simulink model "ringBufferPitchV2"  (R2021a)
settings: Solver=VariableStepAuto  StartTime=0.0  StopTime=10.0  RelTol=1e-3
libraries: hdlsllib x2
settings Model: Creator=Connor Watz  LastModifiedBy=Connor Watz

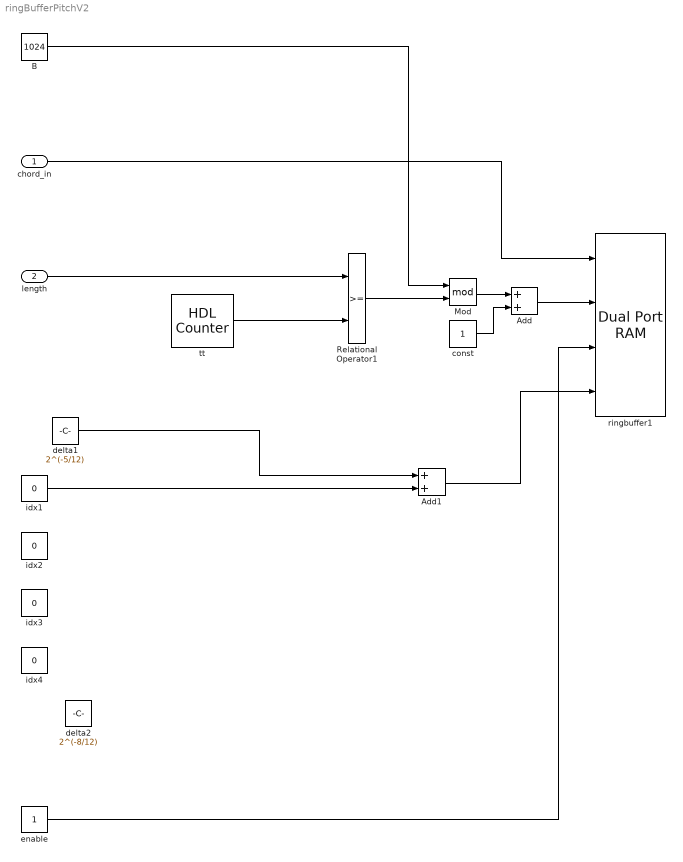
== system ringBufferPitchV2 ==
  chord_in : Inport
  length : Inport  Port=2
  Add : Sum
  Add1 : Sum
  B : Constant  Value=1024  SampleTime=-1
  Mod : Math  Operator=mod  SaturateOnIntegerOverflow=on
  Relational Operator1 : RelationalOperator  OutDataTypeStr=boolean  RndMeth=Nearest
  const : Constant
  delta1 : Constant  Value=2^(-5/12)
  delta2 : Constant  Value=2^(-8/12)
  enable : Constant
  idx{1..4} (4 alike) : Constant  Value=0
  ringbuffer1 : hdlsllib/HDL RAMs/Dual Port RAM  ram_size=8
      settings: SourceProductBaseCode=SL
  tt : hdlsllib/Sources/HDL Counter  CountType=Count limited  CountInit=0  CountStep=1  CountMax=25  CountFromType=Initial value  CountFrom=0  CountResetPort=off  CountLoadPort=off  CountEnbPort=off  CountDirPort=off  CountHitOutputPort=off  CountDataType=Unsigned  CountWordLen=8  CountFracLen=0  CountSampTime=1
  wires:
  length/1 -> Relational Operator1/1
  tt/1 -> Relational Operator1/2
  Relational Operator1/1 -> Mod/2
  B/1 -> Mod/1
  Mod/1 -> Add/1
  Add/1 -> ringbuffer1/2
  const/1 -> Add/2
  enable/1 -> ringbuffer1/3
  idx1/1 -> Add1/2
  delta1/1 -> Add1/1
  Add1/1 -> ringbuffer1/4
  chord_in/1 -> ringbuffer1/1
